simulink library "JointHandler"  (R2017a)
settings: Solver=VariableStepAuto  StartTime=0.0  StopTime=10.0  RelTol=1e-3
values from neighbouring files (symbols this model uses):
  JointControlConfigLHFE = 1245.0    [ModelDictionary.sldd]
  JointControlConfigLKFE = 1245.0    [ModelDictionary.sldd]
  JointControlConfigRHFE = 1245.0    [ModelDictionary.sldd]
  JointControlConfigRKFE = 1245.0    [ModelDictionary.sldd]
undefined symbols (not defined in the file or in its folder): JointCommand
libraries: ConversionsLibrary x8, VariousLibrary x5
settings Model: Creator=march  LastModifiedBy=phil

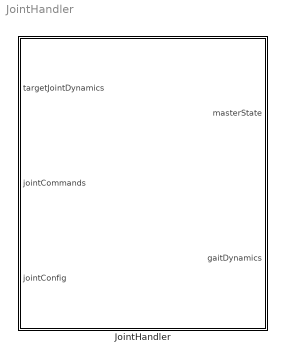
== system JointHandler ==
  JointHandler : Subsystem

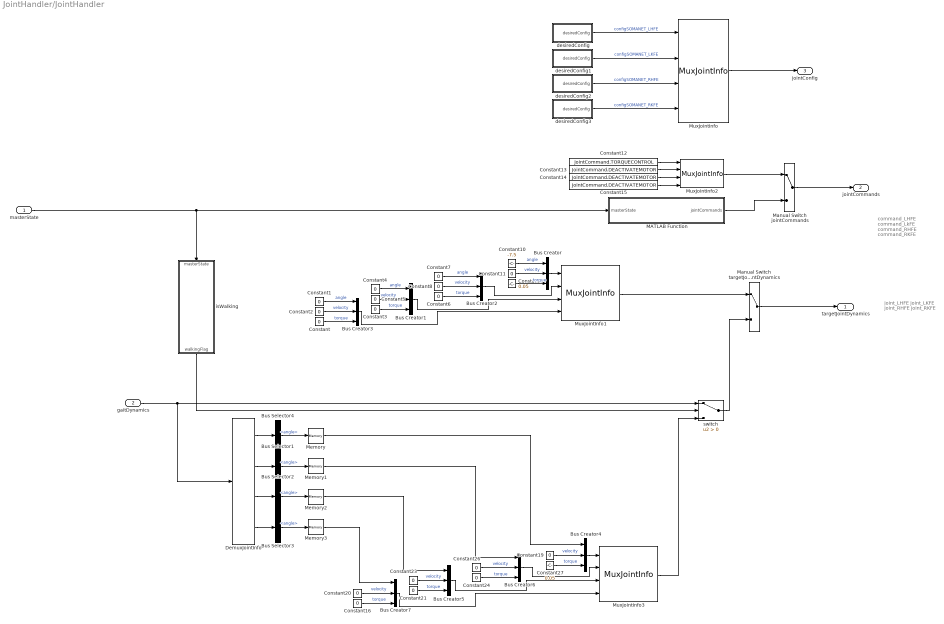
== system JointHandler/JointHandler ==
  note: joint_LHFE
      | joint_LKFE
      | joint_RHFE
      | joint_RKFE
  note: command_LHFE
      | command_LkFE
      | command_RHFE
      | command_RKFE
  masterState : Inport
  gaitDynamics : Inport  Port=2  OutDataTypeStr=Bus: JointDynamics
  Bus Creator{,1..7} (8 alike) : BusCreator  Inputs=3  OutDataTypeStr=Bus: JointDynamics  NonVirtualBus=on
  Bus Selector{1..4} (4 alike) : BusSelector  OutputSignals=angle
  Constant{,1..8,11,16,19..21,23..24,26} (17 alike) : Constant  Value=0
  Constant10 : Constant  Value=-7.5
  Constant12 : Constant  Value=JointCommand.TORQUECONTROL
  Constant13 : Constant  Value=JointCommand.DEACTIVATEMOTOR
  Constant14 : Constant  Value=JointCommand.DEACTIVATEMOTOR
  Constant15 : Constant  Value=JointCommand.DEACTIVATEMOTOR
  Constant27 : Constant  Value=0.05
  Constant9 : Constant  Value=0.05
  DemuxJointInfo : VariousLibrary/DemuxJointInfo
  MATLAB Function : MATLAB Function  TreatAsAtomicUnit=on
  Manual Switch jointCommands : ManualSwitch
  Manual Switch targetJointDynamics : ManualSwitch
  Memory{,1..3} (4 alike) : Memory
  MuxJointInfo{,1..3} (4 alike) : VariousLibrary/MuxJointInfo
  desiredConfig : Subsystem
  desiredConfig1 : Subsystem
  desiredConfig2 : Subsystem
  desiredConfig3 : Subsystem
  isWalking : MATLAB Function  TreatAsAtomicUnit=on
  switch : Switch  Criteria=u2 > Threshold
  targetJointDynamics : Outport  OutDataTypeStr=Bus: JointDynamics  PortDimensions=[1 4]
  jointCommands : Outport  Port=2  OutDataTypeStr=Enum: JointCommand  PortDimensions=[1 4]
  jointConfig : Outport  Port=3  OutDataTypeStr=Bus: JointControlConfig  PortDimensions=[1 4]
  wires:
  switch/1 -> Manual Switch targetJointDynamics/2
  isWalking/1(walkingFlag) -> switch/2
  Memory/1 -> Bus Creator4/1
  Memory1/1 -> Bus Creator6/1
  Memory2/1 -> Bus Creator5/1
  Memory3/1 -> Bus Creator7/1
  Constant24/1 -> Bus Creator6/3  "torque"
  Constant23/1 -> Bus Creator5/2  "velocity"
  Constant16/1 -> Bus Creator7/3  "torque"
  Constant20/1 -> Bus Creator7/2  "velocity"
  Bus Creator6/1 -> MuxJointInfo3/2
  Bus Creator7/1 -> MuxJointInfo3/4
  Bus Creator5/1 -> MuxJointInfo3/3
  Constant19/1 -> Bus Creator4/2  "velocity"
  Bus Creator4/1 -> MuxJointInfo3/1
  Constant21/1 -> Bus Creator5/3  "torque"
  Constant27/1 -> Bus Creator4/3  "torque"
  Constant26/1 -> Bus Creator6/2  "velocity"
  Bus Selector3/1 -> Memory3/1  "<angle>"
  Bus Selector2/1 -> Memory2/1  "<angle>"
  Bus Selector1/1 -> Memory1/1  "<angle>"
  Bus Selector4/1 -> Memory/1  "<angle>"
  DemuxJointInfo/4 -> Bus Selector3/1
  DemuxJointInfo/3 -> Bus Selector2/1
  DemuxJointInfo/2 -> Bus Selector1/1
  DemuxJointInfo/1 -> Bus Selector4/1
  MuxJointInfo3/1 -> switch/3
  gaitDynamics/1 -> switch/1, DemuxJointInfo/1
  Manual Switch targetJointDynamics/1 -> targetJointDynamics/1
  MATLAB Function/1(jointCommands) -> Manual Switch jointCommands/2
  masterState/1 -> isWalking/1(masterState), MATLAB Function/1(masterState)
  MuxJointInfo2/1 -> Manual Switch jointCommands/1
  Constant13/1 -> MuxJointInfo2/2
  Constant14/1 -> MuxJointInfo2/3
  Constant15/1 -> MuxJointInfo2/4
  Constant12/1 -> MuxJointInfo2/1
  Constant9/1 -> Bus Creator/3  "torque"
  Constant11/1 -> Bus Creator/2  "velocity"
  Constant10/1 -> Bus Creator/1  "angle"
  Constant6/1 -> Bus Creator2/3  "torque"
  Constant8/1 -> Bus Creator2/2  "velocity"
  Constant7/1 -> Bus Creator2/1  "angle"
  Constant3/1 -> Bus Creator1/3  "torque"
  Constant5/1 -> Bus Creator1/2  "velocity"
  Constant4/1 -> Bus Creator1/1  "angle"
  Constant/1 -> Bus Creator3/3  "torque"
  Constant2/1 -> Bus Creator3/2  "velocity"
  Constant1/1 -> Bus Creator3/1  "angle"
  Bus Creator2/1 -> MuxJointInfo1/2
  Bus Creator1/1 -> MuxJointInfo1/3
  Bus Creator3/1 -> MuxJointInfo1/4
  Bus Creator/1 -> MuxJointInfo1/1
  MuxJointInfo1/1 -> Manual Switch targetJointDynamics/1
  Manual Switch jointCommands/1 -> jointCommands/1
  MuxJointInfo/1 -> jointConfig/1
  desiredConfig3/1(desiredConfig) -> MuxJointInfo/4  "configSOMANET_RKFE"
  desiredConfig2/1(desiredConfig) -> MuxJointInfo/3  "configSOMANET_RHFE"
  desiredConfig/1(desiredConfig) -> MuxJointInfo/1  "configSOMANET_LHFE"
  desiredConfig1/1(desiredConfig) -> MuxJointInfo/2  "configSOMANET_LKFE"

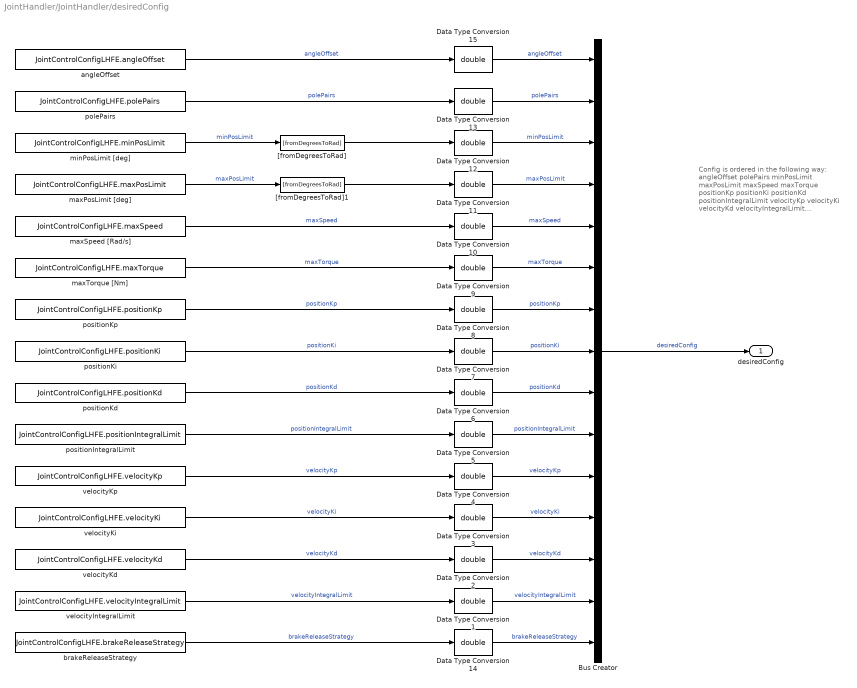
== system JointHandler/JointHandler/desiredConfig ==
  note: Config is ordered in the following way:
      | angleOffset
      | polePairs
      | minPosLimit
      | maxPosLimit
      | maxSpeed
      | maxTorque
      | positionKp
      | positionKi
      | positionKd
      | positionIntegralLimit
      | velocityKp
      | velocityKi
      | velocityKd
      | velocityIntegralLimit
      | brakeReleaseStrategy
  Bus Creator : BusCreator  Inputs=15  OutDataTypeStr=Bus: JointControlConfig  NonVirtualBus=on
  Data Type Conversion{1..15} (15 alike) : DataTypeConversion  OutDataTypeStr=double  RndMeth=Nearest
  "[fromDegreesToRad]" : ConversionsLibrary/[fromDegreesToRad]
  "[fromDegreesToRad]1" : ConversionsLibrary/[fromDegreesToRad]
  angleOffset : Constant  Value=JointControlConfigLHFE.angleOffset  OutDataTypeStr=int32
  brakeReleaseStrategy : Constant  Value=JointControlConfigLHFE.brakeReleaseStrategy  OutDataTypeStr=int32
  maxPosLimit [deg] : Constant  Value=JointControlConfigLHFE.maxPosLimit  OutDataTypeStr=int32
  maxSpeed [Rad/s] : Constant  Value=JointControlConfigLHFE.maxSpeed  OutDataTypeStr=int32
  maxTorque [Nm] : Constant  Value=JointControlConfigLHFE.maxTorque  OutDataTypeStr=int32
  minPosLimit [deg] : Constant  Value=JointControlConfigLHFE.minPosLimit  OutDataTypeStr=int32
  polePairs : Constant  Value=JointControlConfigLHFE.polePairs  OutMin=[0]  OutDataTypeStr=int32
  positionIntegralLimit : Constant  Value=JointControlConfigLHFE.positionIntegralLimit  OutDataTypeStr=int32
  positionKd : Constant  Value=JointControlConfigLHFE.positionKd  OutDataTypeStr=int32
  positionKi : Constant  Value=JointControlConfigLHFE.positionKi  OutDataTypeStr=int32
  positionKp : Constant  Value=JointControlConfigLHFE.positionKp  OutDataTypeStr=int32
  velocityIntegralLimit : Constant  Value=JointControlConfigLHFE.velocityIntegralLimit  OutDataTypeStr=int32
  velocityKd : Constant  Value=JointControlConfigLHFE.velocityKd  OutDataTypeStr=int32
  velocityKi : Constant  Value=JointControlConfigLHFE.velocityKi  OutDataTypeStr=int32
  velocityKp : Constant  Value=JointControlConfigLHFE.velocityKp  OutDataTypeStr=int32
  desiredConfig : Outport  OutDataTypeStr=Bus: JointControlConfig
  wires:
  minPosLimit [deg]/1 -> "[fromDegreesToRad]"/1  "minPosLimit"
  maxPosLimit [deg]/1 -> "[fromDegreesToRad]1"/1  "maxPosLimit"
  Data Type Conversion14/1 -> Bus Creator/15  "brakeReleaseStrategy"
  Data Type Conversion1/1 -> Bus Creator/14  "velocityIntegralLimit"
  Data Type Conversion2/1 -> Bus Creator/13  "velocityKd"
  Data Type Conversion3/1 -> Bus Creator/12  "velocityKi"
  Data Type Conversion4/1 -> Bus Creator/11  "velocityKp"
  Data Type Conversion5/1 -> Bus Creator/10  "positionIntegralLimit"
  Data Type Conversion6/1 -> Bus Creator/9  "positionKd"
  Data Type Conversion7/1 -> Bus Creator/8  "positionKi"
  Data Type Conversion8/1 -> Bus Creator/7  "positionKp"
  Data Type Conversion9/1 -> Bus Creator/6  "maxTorque"
  Data Type Conversion10/1 -> Bus Creator/5  "maxSpeed"
  Data Type Conversion11/1 -> Bus Creator/4  "maxPosLimit"
  Data Type Conversion12/1 -> Bus Creator/3  "minPosLimit"
  Data Type Conversion13/1 -> Bus Creator/2  "polePairs"
  Data Type Conversion15/1 -> Bus Creator/1  "angleOffset"
  Bus Creator/1 -> desiredConfig/1  "desiredConfig"
  velocityKd/1 -> Data Type Conversion2/1  "velocityKd"
  velocityKi/1 -> Data Type Conversion3/1  "velocityKi"
  velocityKp/1 -> Data Type Conversion4/1  "velocityKp"
  positionKd/1 -> Data Type Conversion6/1  "positionKd"
  positionKi/1 -> Data Type Conversion7/1  "positionKi"
  positionKp/1 -> Data Type Conversion8/1  "positionKp"
  maxTorque [Nm]/1 -> Data Type Conversion9/1  "maxTorque"
  velocityIntegralLimit/1 -> Data Type Conversion1/1  "velocityIntegralLimit"
  angleOffset/1 -> Data Type Conversion15/1  "angleOffset"
  brakeReleaseStrategy/1 -> Data Type Conversion14/1  "brakeReleaseStrategy"
  positionIntegralLimit/1 -> Data Type Conversion5/1  "positionIntegralLimit"
  polePairs/1 -> Data Type Conversion13/1  "polePairs"
  maxSpeed [Rad/s]/1 -> Data Type Conversion10/1  "maxSpeed"
  "[fromDegreesToRad]"/1 -> Data Type Conversion12/1
  "[fromDegreesToRad]1"/1 -> Data Type Conversion11/1

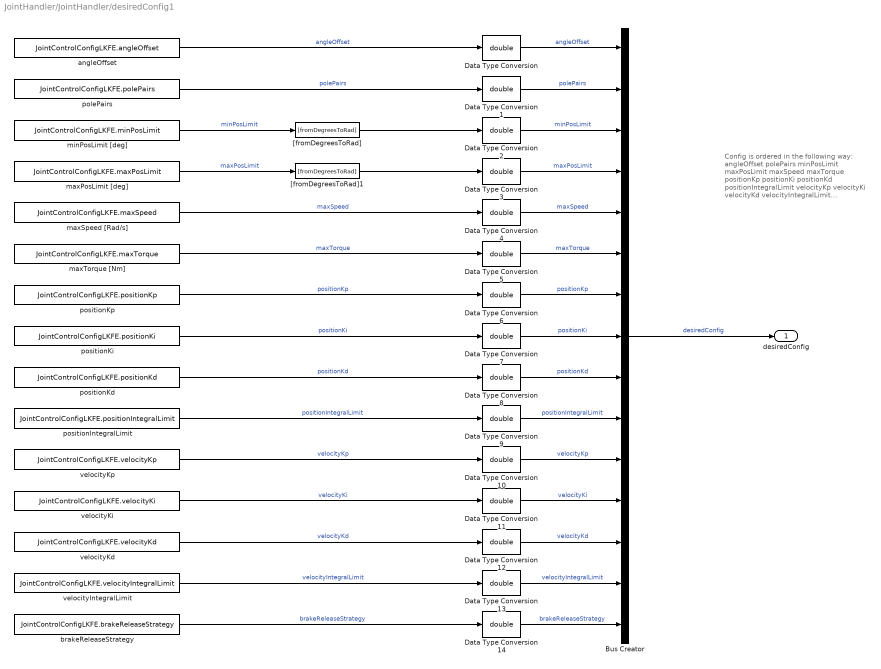
== system JointHandler/JointHandler/desiredConfig1 ==
  note: Config is ordered in the following way:
      | angleOffset
      | polePairs
      | minPosLimit
      | maxPosLimit
      | maxSpeed
      | maxTorque
      | positionKp
      | positionKi
      | positionKd
      | positionIntegralLimit
      | velocityKp
      | velocityKi
      | velocityKd
      | velocityIntegralLimit
      | brakeReleaseStrategy
  Bus Creator : BusCreator  Inputs=15  OutDataTypeStr=Bus: JointControlConfig  NonVirtualBus=on
  Data Type Conversion{,1..14} (15 alike) : DataTypeConversion  OutDataTypeStr=double  RndMeth=Nearest
  "[fromDegreesToRad]" : ConversionsLibrary/[fromDegreesToRad]
  "[fromDegreesToRad]1" : ConversionsLibrary/[fromDegreesToRad]
  angleOffset : Constant  Value=JointControlConfigLKFE.angleOffset  OutDataTypeStr=int32
  brakeReleaseStrategy : Constant  Value=JointControlConfigLKFE.brakeReleaseStrategy  OutDataTypeStr=int32
  maxPosLimit [deg] : Constant  Value=JointControlConfigLKFE.maxPosLimit  OutDataTypeStr=int32
  maxSpeed [Rad/s] : Constant  Value=JointControlConfigLKFE.maxSpeed  OutDataTypeStr=int32
  maxTorque [Nm] : Constant  Value=JointControlConfigLKFE.maxTorque  OutDataTypeStr=int32
  minPosLimit [deg] : Constant  Value=JointControlConfigLKFE.minPosLimit  OutDataTypeStr=int32
  polePairs : Constant  Value=JointControlConfigLKFE.polePairs  OutMin=[0]  OutDataTypeStr=int32
  positionIntegralLimit : Constant  Value=JointControlConfigLKFE.positionIntegralLimit  OutDataTypeStr=int32
  positionKd : Constant  Value=JointControlConfigLKFE.positionKd  OutDataTypeStr=int32
  positionKi : Constant  Value=JointControlConfigLKFE.positionKi  OutDataTypeStr=int32
  positionKp : Constant  Value=JointControlConfigLKFE.positionKp  OutDataTypeStr=int32
  velocityIntegralLimit : Constant  Value=JointControlConfigLKFE.velocityIntegralLimit  OutDataTypeStr=int32
  velocityKd : Constant  Value=JointControlConfigLKFE.velocityKd  OutDataTypeStr=int32
  velocityKi : Constant  Value=JointControlConfigLKFE.velocityKi  OutDataTypeStr=int32
  velocityKp : Constant  Value=JointControlConfigLKFE.velocityKp  OutDataTypeStr=int32
  desiredConfig : Outport  OutDataTypeStr=Bus: JointControlConfig
  wires:
  minPosLimit [deg]/1 -> "[fromDegreesToRad]"/1  "minPosLimit"
  maxPosLimit [deg]/1 -> "[fromDegreesToRad]1"/1  "maxPosLimit"
  Data Type Conversion14/1 -> Bus Creator/15  "brakeReleaseStrategy"
  Data Type Conversion13/1 -> Bus Creator/14  "velocityIntegralLimit"
  Data Type Conversion12/1 -> Bus Creator/13  "velocityKd"
  Data Type Conversion11/1 -> Bus Creator/12  "velocityKi"
  Data Type Conversion10/1 -> Bus Creator/11  "velocityKp"
  Data Type Conversion9/1 -> Bus Creator/10  "positionIntegralLimit"
  Data Type Conversion8/1 -> Bus Creator/9  "positionKd"
  Data Type Conversion7/1 -> Bus Creator/8  "positionKi"
  Data Type Conversion6/1 -> Bus Creator/7  "positionKp"
  Data Type Conversion5/1 -> Bus Creator/6  "maxTorque"
  Data Type Conversion4/1 -> Bus Creator/5  "maxSpeed"
  Data Type Conversion3/1 -> Bus Creator/4  "maxPosLimit"
  Data Type Conversion2/1 -> Bus Creator/3  "minPosLimit"
  Data Type Conversion1/1 -> Bus Creator/2  "polePairs"
  Data Type Conversion/1 -> Bus Creator/1  "angleOffset"
  Bus Creator/1 -> desiredConfig/1  "desiredConfig"
  velocityKd/1 -> Data Type Conversion12/1  "velocityKd"
  velocityKi/1 -> Data Type Conversion11/1  "velocityKi"
  velocityKp/1 -> Data Type Conversion10/1  "velocityKp"
  positionKd/1 -> Data Type Conversion8/1  "positionKd"
  positionKi/1 -> Data Type Conversion7/1  "positionKi"
  positionKp/1 -> Data Type Conversion6/1  "positionKp"
  maxTorque [Nm]/1 -> Data Type Conversion5/1  "maxTorque"
  velocityIntegralLimit/1 -> Data Type Conversion13/1  "velocityIntegralLimit"
  angleOffset/1 -> Data Type Conversion/1  "angleOffset"
  brakeReleaseStrategy/1 -> Data Type Conversion14/1  "brakeReleaseStrategy"
  positionIntegralLimit/1 -> Data Type Conversion9/1  "positionIntegralLimit"
  polePairs/1 -> Data Type Conversion1/1  "polePairs"
  maxSpeed [Rad/s]/1 -> Data Type Conversion4/1  "maxSpeed"
  "[fromDegreesToRad]"/1 -> Data Type Conversion2/1
  "[fromDegreesToRad]1"/1 -> Data Type Conversion3/1

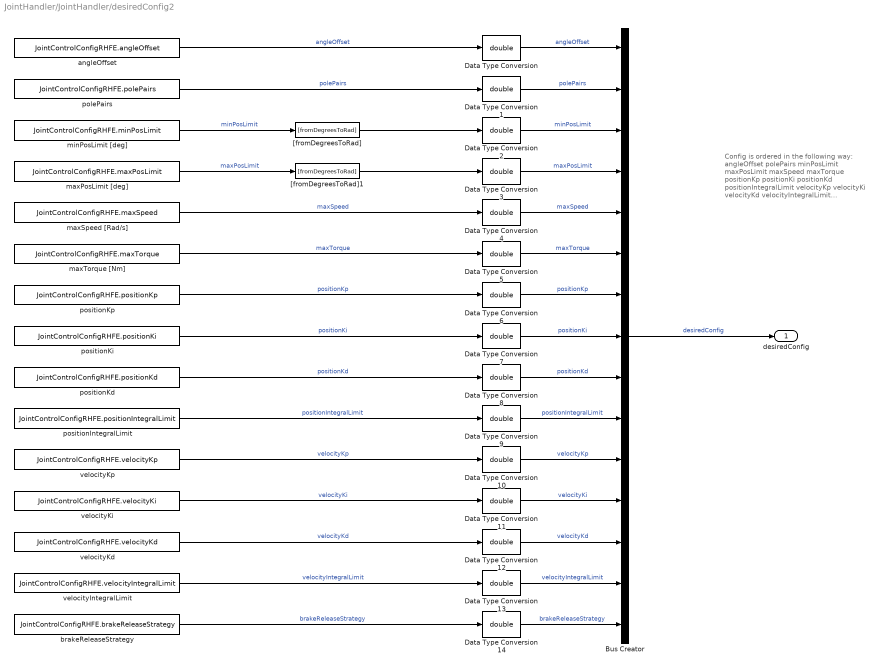
== system JointHandler/JointHandler/desiredConfig2 ==
  note: Config is ordered in the following way:
      | angleOffset
      | polePairs
      | minPosLimit
      | maxPosLimit
      | maxSpeed
      | maxTorque
      | positionKp
      | positionKi
      | positionKd
      | positionIntegralLimit
      | velocityKp
      | velocityKi
      | velocityKd
      | velocityIntegralLimit
      | brakeReleaseStrategy
  Bus Creator : BusCreator  Inputs=15  OutDataTypeStr=Bus: JointControlConfig  NonVirtualBus=on
  Data Type Conversion{,1..14} (15 alike) : DataTypeConversion  OutDataTypeStr=double  RndMeth=Nearest
  "[fromDegreesToRad]" : ConversionsLibrary/[fromDegreesToRad]
  "[fromDegreesToRad]1" : ConversionsLibrary/[fromDegreesToRad]
  angleOffset : Constant  Value=JointControlConfigRHFE.angleOffset  OutDataTypeStr=int32
  brakeReleaseStrategy : Constant  Value=JointControlConfigRHFE.brakeReleaseStrategy  OutDataTypeStr=int32
  maxPosLimit [deg] : Constant  Value=JointControlConfigRHFE.maxPosLimit  OutDataTypeStr=int32
  maxSpeed [Rad/s] : Constant  Value=JointControlConfigRHFE.maxSpeed  OutDataTypeStr=int32
  maxTorque [Nm] : Constant  Value=JointControlConfigRHFE.maxTorque  OutDataTypeStr=int32
  minPosLimit [deg] : Constant  Value=JointControlConfigRHFE.minPosLimit  OutDataTypeStr=int32
  polePairs : Constant  Value=JointControlConfigRHFE.polePairs  OutMin=[0]  OutDataTypeStr=int32
  positionIntegralLimit : Constant  Value=JointControlConfigRHFE.positionIntegralLimit  OutDataTypeStr=int32
  positionKd : Constant  Value=JointControlConfigRHFE.positionKd  OutDataTypeStr=int32
  positionKi : Constant  Value=JointControlConfigRHFE.positionKi  OutDataTypeStr=int32
  positionKp : Constant  Value=JointControlConfigRHFE.positionKp  OutDataTypeStr=int32
  velocityIntegralLimit : Constant  Value=JointControlConfigRHFE.velocityIntegralLimit  OutDataTypeStr=int32
  velocityKd : Constant  Value=JointControlConfigRHFE.velocityKd  OutDataTypeStr=int32
  velocityKi : Constant  Value=JointControlConfigRHFE.velocityKi  OutDataTypeStr=int32
  velocityKp : Constant  Value=JointControlConfigRHFE.velocityKp  OutDataTypeStr=int32
  desiredConfig : Outport  OutDataTypeStr=Bus: JointControlConfig
  wires:
  minPosLimit [deg]/1 -> "[fromDegreesToRad]"/1  "minPosLimit"
  maxPosLimit [deg]/1 -> "[fromDegreesToRad]1"/1  "maxPosLimit"
  Data Type Conversion14/1 -> Bus Creator/15  "brakeReleaseStrategy"
  Data Type Conversion13/1 -> Bus Creator/14  "velocityIntegralLimit"
  Data Type Conversion12/1 -> Bus Creator/13  "velocityKd"
  Data Type Conversion11/1 -> Bus Creator/12  "velocityKi"
  Data Type Conversion10/1 -> Bus Creator/11  "velocityKp"
  Data Type Conversion9/1 -> Bus Creator/10  "positionIntegralLimit"
  Data Type Conversion8/1 -> Bus Creator/9  "positionKd"
  Data Type Conversion7/1 -> Bus Creator/8  "positionKi"
  Data Type Conversion6/1 -> Bus Creator/7  "positionKp"
  Data Type Conversion5/1 -> Bus Creator/6  "maxTorque"
  Data Type Conversion4/1 -> Bus Creator/5  "maxSpeed"
  Data Type Conversion3/1 -> Bus Creator/4  "maxPosLimit"
  Data Type Conversion2/1 -> Bus Creator/3  "minPosLimit"
  Data Type Conversion1/1 -> Bus Creator/2  "polePairs"
  Data Type Conversion/1 -> Bus Creator/1  "angleOffset"
  Bus Creator/1 -> desiredConfig/1  "desiredConfig"
  velocityKd/1 -> Data Type Conversion12/1  "velocityKd"
  velocityKi/1 -> Data Type Conversion11/1  "velocityKi"
  velocityKp/1 -> Data Type Conversion10/1  "velocityKp"
  positionKd/1 -> Data Type Conversion8/1  "positionKd"
  positionKi/1 -> Data Type Conversion7/1  "positionKi"
  positionKp/1 -> Data Type Conversion6/1  "positionKp"
  maxTorque [Nm]/1 -> Data Type Conversion5/1  "maxTorque"
  velocityIntegralLimit/1 -> Data Type Conversion13/1  "velocityIntegralLimit"
  angleOffset/1 -> Data Type Conversion/1  "angleOffset"
  brakeReleaseStrategy/1 -> Data Type Conversion14/1  "brakeReleaseStrategy"
  positionIntegralLimit/1 -> Data Type Conversion9/1  "positionIntegralLimit"
  polePairs/1 -> Data Type Conversion1/1  "polePairs"
  maxSpeed [Rad/s]/1 -> Data Type Conversion4/1  "maxSpeed"
  "[fromDegreesToRad]"/1 -> Data Type Conversion2/1
  "[fromDegreesToRad]1"/1 -> Data Type Conversion3/1

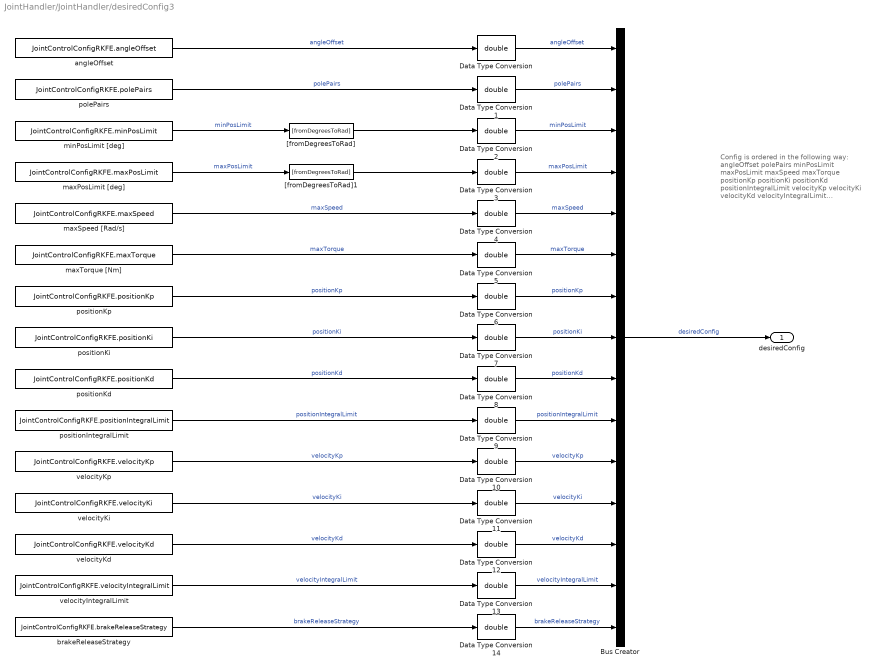
== system JointHandler/JointHandler/desiredConfig3 ==
  note: Config is ordered in the following way:
      | angleOffset
      | polePairs
      | minPosLimit
      | maxPosLimit
      | maxSpeed
      | maxTorque
      | positionKp
      | positionKi
      | positionKd
      | positionIntegralLimit
      | velocityKp
      | velocityKi
      | velocityKd
      | velocityIntegralLimit
      | brakeReleaseStrategy
  Bus Creator : BusCreator  Inputs=15  OutDataTypeStr=Bus: JointControlConfig  NonVirtualBus=on
  Data Type Conversion{,1..14} (15 alike) : DataTypeConversion  OutDataTypeStr=double  RndMeth=Nearest
  "[fromDegreesToRad]" : ConversionsLibrary/[fromDegreesToRad]
  "[fromDegreesToRad]1" : ConversionsLibrary/[fromDegreesToRad]
  angleOffset : Constant  Value=JointControlConfigRKFE.angleOffset  OutDataTypeStr=int32
  brakeReleaseStrategy : Constant  Value=JointControlConfigRKFE.brakeReleaseStrategy  OutDataTypeStr=int32
  maxPosLimit [deg] : Constant  Value=JointControlConfigRKFE.maxPosLimit  OutDataTypeStr=int32
  maxSpeed [Rad/s] : Constant  Value=JointControlConfigRKFE.maxSpeed  OutDataTypeStr=int32
  maxTorque [Nm] : Constant  Value=JointControlConfigRKFE.maxTorque  OutDataTypeStr=int32
  minPosLimit [deg] : Constant  Value=JointControlConfigRKFE.minPosLimit  OutDataTypeStr=int32
  polePairs : Constant  Value=JointControlConfigRKFE.polePairs  OutMin=[0]  OutDataTypeStr=int32
  positionIntegralLimit : Constant  Value=JointControlConfigRKFE.positionIntegralLimit  OutDataTypeStr=int32
  positionKd : Constant  Value=JointControlConfigRKFE.positionKd  OutDataTypeStr=int32
  positionKi : Constant  Value=JointControlConfigRKFE.positionKi  OutDataTypeStr=int32
  positionKp : Constant  Value=JointControlConfigRKFE.positionKp  OutDataTypeStr=int32
  velocityIntegralLimit : Constant  Value=JointControlConfigRKFE.velocityIntegralLimit  OutDataTypeStr=int32
  velocityKd : Constant  Value=JointControlConfigRKFE.velocityKd  OutDataTypeStr=int32
  velocityKi : Constant  Value=JointControlConfigRKFE.velocityKi  OutDataTypeStr=int32
  velocityKp : Constant  Value=JointControlConfigRKFE.velocityKp  OutDataTypeStr=int32
  desiredConfig : Outport  OutDataTypeStr=Bus: JointControlConfig
  wires:
  minPosLimit [deg]/1 -> "[fromDegreesToRad]"/1  "minPosLimit"
  maxPosLimit [deg]/1 -> "[fromDegreesToRad]1"/1  "maxPosLimit"
  Data Type Conversion14/1 -> Bus Creator/15  "brakeReleaseStrategy"
  Data Type Conversion13/1 -> Bus Creator/14  "velocityIntegralLimit"
  Data Type Conversion12/1 -> Bus Creator/13  "velocityKd"
  Data Type Conversion11/1 -> Bus Creator/12  "velocityKi"
  Data Type Conversion10/1 -> Bus Creator/11  "velocityKp"
  Data Type Conversion9/1 -> Bus Creator/10  "positionIntegralLimit"
  Data Type Conversion8/1 -> Bus Creator/9  "positionKd"
  Data Type Conversion7/1 -> Bus Creator/8  "positionKi"
  Data Type Conversion6/1 -> Bus Creator/7  "positionKp"
  Data Type Conversion5/1 -> Bus Creator/6  "maxTorque"
  Data Type Conversion4/1 -> Bus Creator/5  "maxSpeed"
  Data Type Conversion3/1 -> Bus Creator/4  "maxPosLimit"
  Data Type Conversion2/1 -> Bus Creator/3  "minPosLimit"
  Data Type Conversion1/1 -> Bus Creator/2  "polePairs"
  Data Type Conversion/1 -> Bus Creator/1  "angleOffset"
  Bus Creator/1 -> desiredConfig/1  "desiredConfig"
  velocityKd/1 -> Data Type Conversion12/1  "velocityKd"
  velocityKi/1 -> Data Type Conversion11/1  "velocityKi"
  velocityKp/1 -> Data Type Conversion10/1  "velocityKp"
  positionKd/1 -> Data Type Conversion8/1  "positionKd"
  positionKi/1 -> Data Type Conversion7/1  "positionKi"
  positionKp/1 -> Data Type Conversion6/1  "positionKp"
  maxTorque [Nm]/1 -> Data Type Conversion5/1  "maxTorque"
  velocityIntegralLimit/1 -> Data Type Conversion13/1  "velocityIntegralLimit"
  angleOffset/1 -> Data Type Conversion/1  "angleOffset"
  brakeReleaseStrategy/1 -> Data Type Conversion14/1  "brakeReleaseStrategy"
  positionIntegralLimit/1 -> Data Type Conversion9/1  "positionIntegralLimit"
  polePairs/1 -> Data Type Conversion1/1  "polePairs"
  maxSpeed [Rad/s]/1 -> Data Type Conversion4/1  "maxSpeed"
  "[fromDegreesToRad]"/1 -> Data Type Conversion2/1
  "[fromDegreesToRad]1"/1 -> Data Type Conversion3/1

== matlab function JointHandler/MATLAB Function ==
  data: masterState input; jointCommands output
function jointCommands = getJointCommandsFromState(masterState)
jointCommands = [ JointCommand.DEACTIVATEMOTOR JointCommand.DEACTIVATEMOTOR JointCommand.DEACTIVATEMOTOR JointCommand.DEACTIVATEMOTOR];
end

== matlab function JointHandler/isWalking ==
  data: masterState input; walkingFlag output
function walkingFlag = isWalking(masterState)
% This function should determine whether the exoskeleton is walking. If not
% the flag is set and the current position is hold.
if masterState == Exoskeleton.HOLDSIT || masterState == Exoskeleton.HOLDSTAND
    walkingFlag = 0;
else
    walkingFlag = 1;
end
